simulink model "mod_16QAM"  (Simulink 10.3)
settings: Solver=FixedStepDiscrete  StartTime=0.0  StopTime=10  RelTol=1e-3  EnableMultiTasking=on
InitFcn:
  | mod_16QAM_m
values from neighbouring files (symbols this model uses):
  f0 = 1e4    (= 10000)    [mod_16QAM_m.m]
  frame = 128    [mod_16QAM_m.m]
  N_samples = K * of    (= 120)    [mod_16QAM_m.m]
  Tc = 1/fc    (= 2.26757369615e-05)    [mod_16QAM_m.m]
libraries: dspsrcs4 x2, commfilt2 x2, commrandsrc3 x1, commdigbbndam3 x1
settings Model: Creator=Francesco  LastModifiedBy=pierr
settings DataIOCC: LimitDataPoints=on
settings DebuggingCC: SolverPrmCheckMsg=warning
settings ConfigComp: CovExternalEMLEnable=on

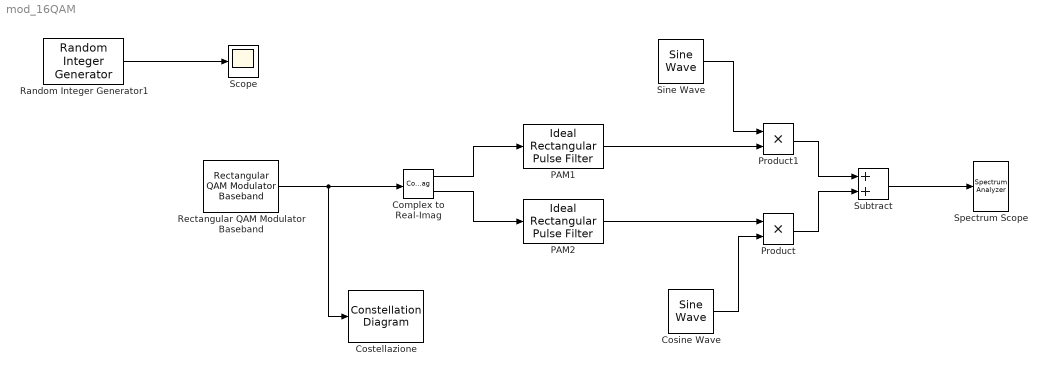
== system mod_16QAM ==
  Complex to Real-Imag : ComplexToRealImag
  Cosine Wave : dspsrcs4/Sine Wave  Amplitude=1  Frequency=f0  Phase=pi/2  SampleMode=Discrete  OutComplex=Real  CompMethod=Trigonometric fcn  TableSize=Speed  SampleTime=Tc  SamplesPerFrame=N_samples*frame  ResetState=Restart at time zero  OutputFrames=on  dataType=double  wordLen=16  udDataType=sfix(16)  fracBitsMode=Best precision  numFracBits=15  OutDataTypeStr=double  LastOutDataTypeStr=double
  Costellazione : ConstellationDiagram  Tag=ScatterPlot
  PAM1 : commfilt2/Ideal Rectangular Pulse Filter  pulseLen=N_samples  pulseDelay=0  InputProcessing=Columns as channels (frame based)  RateOptions=Enforce single-rate processing  sampMode=Frame-based  normCheck=off  normMode=Sum of samples  filterGain=1  saveAsFlag=0  roundingMode=Floor  overflowMode=off  firstCoeffDataTypeStr=Inherit: Same word length as input  firstCoeffMin=[]  firstCoeffMax=[]  firstCoeffLastDataTypeStr=Inherit: Same word length as input  outputDataTypeStr=Inherit: Same as accumulator  outputMin=[]  outputMax=[]  outputLastDataTypeStr=Inherit: Same as accumulator
      settings: SourceProductBaseCode=CM
  PAM2 : commfilt2/Ideal Rectangular Pulse Filter  pulseLen=N_samples  pulseDelay=0  InputProcessing=Columns as channels (frame based)  RateOptions=Enforce single-rate processing  sampMode=Frame-based  normCheck=off  normMode=Sum of samples  filterGain=1  saveAsFlag=0  roundingMode=Floor  overflowMode=off  firstCoeffDataTypeStr=Inherit: Same word length as input  firstCoeffMin=[]  firstCoeffMax=[]  firstCoeffLastDataTypeStr=Inherit: Same word length as input  outputDataTypeStr=Inherit: Same as accumulator  outputMin=[]  outputMax=[]  outputLastDataTypeStr=Inherit: Same as accumulator
      settings: SourceProductBaseCode=CM
  Product : Product  RndMeth=Zero
  Product1 : Product  RndMeth=Zero
  Random Integer Generator1 : commrandsrc3/Random Integer Generator  SetSize=20  SeedSource=Auto  Seed=0  SampleTime=1  SamplesPerFrame=1  OutputDataType=double  SimulateUsing=Interpreted execution
  Rectangular QAM Modulator Baseband : commdigbbndam3/Rectangular QAM Modulator Baseband  M=16  InType=Integer  Enc=Gray  Mapping=[0:15]  PowType=Min. distance between symbols  MinDist=2  AvgPow=1  PeakPow=1  Ph=0  outDtype=double  outWordLen=16  outUDDataType=sfix(16)  outFracLenMode=Best precision  outFracLen=15  outDataTypeStr=double  outLastDataTypeStr=double
  Scope : Scope
  Sine Wave : dspsrcs4/Sine Wave  Amplitude=1  Frequency=f0  Phase=0  SampleMode=Discrete  OutComplex=Real  CompMethod=Trigonometric fcn  TableSize=Speed  SampleTime=Tc  SamplesPerFrame=N_samples*frame  ResetState=Restart at time zero  OutputFrames=on  dataType=double  wordLen=16  udDataType=sfix(16)  fracBitsMode=Best precision  numFracBits=15  OutDataTypeStr=double  LastOutDataTypeStr=double
  Spectrum Scope : SpectrumAnalyzer
  Subtract : Sum
  wires:
  Rectangular QAM Modulator Baseband/1 -> Complex to Real-Imag/1, Costellazione/1
  Complex to Real-Imag/2 -> PAM2/1
  PAM2/1 -> Product/1
  PAM1/1 -> Product1/2
  Complex to Real-Imag/1 -> PAM1/1
  Product1/1 -> Subtract/1
  Product/1 -> Subtract/2
  Subtract/1 -> Spectrum Scope/1
  Sine Wave/1 -> Product1/1
  Cosine Wave/1 -> Product/2
  Random Integer Generator1/1 -> Scope/1
